simulink model "untitled"  (R2025b)
settings: Solver=FixedStepAuto  StartTime=0.0  StopTime=10.0  FixedStep=0.01  RelTol=1e-3
settings Model: Creator=gurkirat  LastModifiedBy=gurkirat

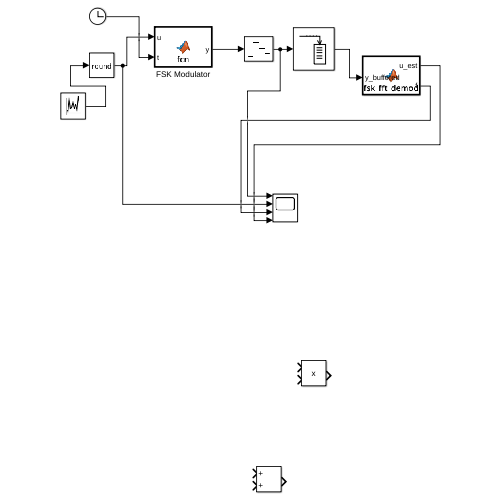
[thumbnail: Simulink's stored preview of the top-level diagram]
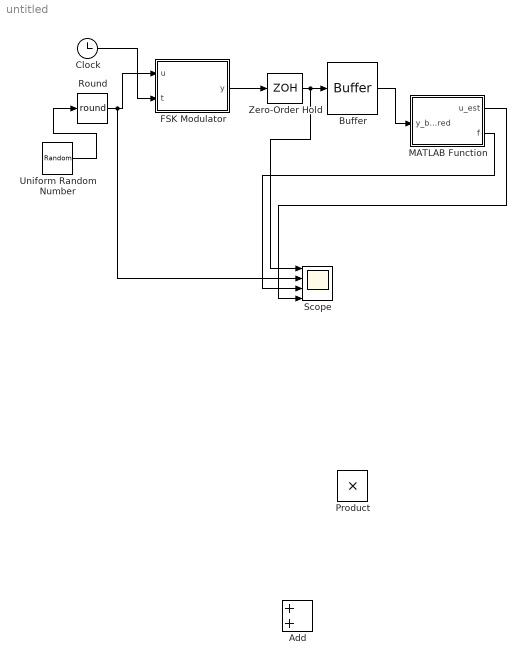
== system untitled ==
  Add : Sum
  Buffer : Buffer  N=50  OutputFrames=off
  Clock : Clock
  FSK Modulator : MATLAB Function  TreatAsAtomicUnit=on
  MATLAB Function : MATLAB Function  TreatAsAtomicUnit=on
  Product : Product
  Round : Rounding  Operator=round
  Scope : Scope  NumInputPorts=4
      settings: ActiveDisplayYMinimum=-9.512580984376088  ActiveDisplayYMaximum=15.099814557122089
  Uniform Random Number : UniformRandomNumber  Minimum=0  Maximum=3  SampleTime=1
  Zero-Order Hold : ZeroOrderHold  SampleTime=.02
  wires:
  Clock/1 -> FSK Modulator/2(t)
  Uniform Random Number/1 -> Round/1
  Round/1 -> Scope/2, FSK Modulator/1(u)
  MATLAB Function/1(u_est) -> Scope/4
  MATLAB Function/2(f) -> Scope/3
  FSK Modulator/1(y) -> Zero-Order Hold/1
  Zero-Order Hold/1 -> Scope/1, Buffer/1
  Buffer/1 -> MATLAB Function/1(y_buffered)

== matlab function untitled/FSK Modulator ==
  data: u input; y output; t input
function y = fcn(u,t)

y = 5*sin(2*5*pi*u*t);

== matlab function untitled/MATLAB Function ==
  data: y_buffered input; u_est output; f output
function [u_est,f] = fsk_fft_demod(y_buffered)
N=length(y_buffered);
Y=fft(y_buffered);
P2=abs(Y/N);
P1=2*P2(1:26);
f=50*(0:25)/50
[max_A,max_idx]=max(P1)

u_est=round((max_idx)/5)
end
